simulink model "Proyecto_Final"  (R2017a)
settings: Solver=ode45  StartTime=0.0  StopTime=inf  FixedStep=0.002  RelTol=1e-4
values from neighbouring files (symbols this model uses):
  b_h = b_eq_h * r_h ^ 2 / R_d ^ 2    (= 28800)    [automatas_matlab.m]
  b_t = b_eq_t * r_t ^ 2 / R_w_t ^ 2    (= 27000)    [automatas_matlab.m]
  b_w_h = 30000    [automatas_matlab.m]
  ba_h = M_h * n_h * w_pos_h    (= 172800)    [automatas_matlab.m]
  ba_t = M_t * n_t * w_pos_t    (= 135000)    [automatas_matlab.m]
  bottom_limit_0 = -22    [automatas_matlab.m]
  bottom_limit_1 = -20    [automatas_matlab.m]
  container_vector = [2, 6, 4, 1, 5, 8, 1, 3, 7, 1, 5, 6]    [automatas_matlab.m]    (also in plot_crane.m = [8, 12, 12, 4, 5, 8, 1, 3]; test_traj.m = [8, 5, 9, 4, 5, 8, 4, 6]; test_trajectories.m = [8, 12, 12, 4, 5, 8, 1, 3, 7, 1, 5, 6])
  g = 9.80665    [automatas_matlab.m]
  h_contenedor = 2.79    [automatas_matlab.m]
  K_w_h = 1800000    [automatas_matlab.m]
  Ksa_h = M_h * n_h * w_pos_h^2    (= 207298.578199)    [automatas_matlab.m]
  Ksa_t = M_t * n_t * w_pos_t^2    (= 123542.570499)    [automatas_matlab.m]
  Ksia_h = M_h * w_pos_h ^ 3    (= 82894.8698367)    [automatas_matlab.m]
  Ksia_t = M_t * w_pos_t ^ 3    (= 45223.0125199)    [automatas_matlab.m]
  lambda = 0.91    [automatas_matlab.m]
  left_limit_0 = -32    [automatas_matlab.m]
  left_limit_1 = -30    [automatas_matlab.m]
  M_h = (J_d + J_m_h * r_h ^ 2)/ R_d ^ 2    (= 48014.2222222)    [automatas_matlab.m]
  m_l = 65000    [automatas_matlab.m]
  m_l_min = 15000    [automatas_matlab.m]
  M_t = m_c + (J_w_t + J_m_t * r_t ^ 2)/ R_w_t ^ 2    (= 59008)    [automatas_matlab.m]
  R_d = 0.75    [automatas_matlab.m]
  r_h = 30    [automatas_matlab.m]
  r_t = 15    [automatas_matlab.m]
  R_w_t = 0.5    [automatas_matlab.m]
  right_limit_0 = 52    [automatas_matlab.m]
  right_limit_1 = 50    [automatas_matlab.m]
  top_limit_0 = 42    [automatas_matlab.m]
  top_limit_1 = 40    [automatas_matlab.m]
  v_max_h_load = 1.5    [automatas_matlab.m]
  v_max_h_unload = 3    [automatas_matlab.m]
  v_max_t = 4    [automatas_matlab.m]
  x_t0 = 0    [automatas_matlab.m]
  y_t0 = 45    [automatas_matlab.m]    (also in crane.m; plot_crane.m; plot_crane_test.m)
  yl0 = h_contenedor + 5    (= 7.79)    [automatas_matlab.m]
undefined symbols (not defined in the file or in its folder): DiscIntNeverNeededParam
libraries: simulink x8, vrlib x1, sldrtlib x1
(part 2 of 2)

== stateflow chart Proyecto_Final/Level_1  ==
  settings: updateMethod=DISCRETE  sampleTime=0.01
  state Level1
    entry:
    go_to_ship = 1;
    to_manual = 0;
    ml = m_l;
    v_max_h = v_max_h_load;
    charged = 1;
    during:
    state Start [parallel]
      entry:
      traj_plt = plot(0, 0, 'r' );
      during:
      settings: executionOrder=4
      state Automatico
        entry:
        pos_ini_ = pos_ini;
        pos_fin_ = pos_fin;
        if go_to_ship == 0
        [pos_ini_, pos_fin_] = get_pos(pos_ini, pos_fin, container_vector);
        end
        [x_traj, y_traj] = get_trajectories(pos_ini_, pos_fin_, charged, container_vector);
        mode = 0;
        hold on
        during:
        %v_h_1 = 0.1;
        %v_t_1 = 0.1;
        state to_ship
          entry:
          to_ship_finished = 0;
          above_trajectory = 0;
          during:
          state Vertical
            entry:
            y_finish = get_y_finish();
            during:
            if y_finish > yl
            v_h_1 = - v_max_h * vertical_gain() ;
            else
            above_trajectory = 1;
            end
            v_t_1 = 0;
          state Diagonal_Up
            entry:
            [vh1_, vt1_] = get_v_up(1, 1);
            during:
            my_gain = get_gains();
            v_h_1 = vh1_ * my_gain;
            v_t_1 = vt1_ * my_gain;
          state Horizontal
            entry:
            during:
            my_gain = get_gains();
            v_h_1 = 0;
            v_t_1 = v_max_t * my_gain;
          state Diagonal_Down
            entry:
            [vh_1, vt_1] = get_v_down(1, 1);
            during:
            my_gain = get_gains();
            v_h_1 = vh_1 * my_gain;
            v_t_1 = vt_1 * my_gain;
          state Stop
            during:
            v_h_1 = 0;
            v_t_1 = 0;
            to_ship_finished = 1;
            go_to_ship = 0;
          (default) -> Level1.Start.Automatico.to_ship.Vertical
          Level1.Start.Automatico.to_ship.Vertical -> Level1.Start.Automatico.to_ship.Diagonal_Up [order 3] : [above_trajectory == 1]
          Level1.Start.Automatico.to_ship.Vertical -> Level1.Start.Automatico.to_ship.Diagonal_Down [order 2] : [xl > x_traj(3)]
          Level1.Start.Automatico.to_ship.Vertical -> Level1.Start.Automatico.to_ship.Diagonal_Up [order 1] : [(yl > (y_finish - 0.1)) && (yl < (y_finish + 0.1))]
          Level1.Start.Automatico.to_ship.Diagonal_Up -> Level1.Start.Automatico.to_ship.Horizontal : [yl >=  y_traj(2)]
          Level1.Start.Automatico.to_ship.Horizontal -> Level1.Start.Automatico.to_ship.Diagonal_Down : [xt > x_traj(3)]
          Level1.Start.Automatico.to_ship.Diagonal_Down -> Level1.Start.Automatico.to_ship.Stop : [xt > x_traj(4) && abs(yl - y_traj(4)) < 2]
        state from_ship
          entry:
          from_ship_finished = 0;
          above_trajectory = 0;
          during:
          state Vertical
            entry:
            y_finish = get_y_finish();
            during:
            if y_finish > yl
            v_h_1 = - v_max_h * vertical_gain();
            else
            above_trajectory = 1;
            end
            v_t_1 = 0;
          state Diagonal_Up
            entry:
            [vh1_, vt1_] = get_v_up_return(1, 1);
            during:
            my_gain = get_gains_return();
            v_h_1 = vh1_ * my_gain;
            v_t_1 = vt1_ * my_gain;
          state Horizontal
            entry:
            during:
            my_gain = get_gains_return();
            v_h_1 = 0;
            v_t_1 = -v_max_t * my_gain;
          state Diagonal_Down
            entry:
            [vh_1, vt_1] = get_v_down_return(1, 1);
            during:
            my_gain = get_gains_return();
            v_h_1 = vh_1 * my_gain;
            v_t_1 = vt_1 * my_gain;
          state Stop
            during:
            v_h_1 = 0;
            v_t_1 = 0;
            from_ship_finished = 1;
            go_to_ship = 1;
          (default) -> Level1.Start.Automatico.from_ship.Vertical
          Level1.Start.Automatico.from_ship.Vertical -> Level1.Start.Automatico.from_ship.Diagonal_Up [order 3] : [above_trajectory == 1]
          Level1.Start.Automatico.from_ship.Vertical -> Level1.Start.Automatico.from_ship.Diagonal_Down [order 2] : [xl < x_traj(2)]
          Level1.Start.Automatico.from_ship.Vertical -> Level1.Start.Automatico.from_ship.Diagonal_Up [order 1] : [(yl > (y_finish - 0.1)) && (yl < (y_finish + 0.1))]
          Level1.Start.Automatico.from_ship.Diagonal_Up -> Level1.Start.Automatico.from_ship.Horizontal : [yl >=  y_traj(3)]
          Level1.Start.Automatico.from_ship.Horizontal -> Level1.Start.Automatico.from_ship.Diagonal_Down : [xt < x_traj(2)]
          Level1.Start.Automatico.from_ship.Diagonal_Down -> Level1.Start.Automatico.from_ship.Stop : [xt < x_traj(1) && abs(yl - y_traj(1)) < 2]
        state Wait
          entry: from_ship_finished = 0;
          to_ship_finished = 0;
          entry:
          during:
          v_h_1 = 0;
          v_t_1 = 0;
        (default) -> Wait
        Wait -> from_ship [order 2] : [go_to_ship == 0 && automatic == 1]
        Wait -> to_ship [order 1] : [go_to_ship == 1 && automatic == 1]
        from_ship -> Wait : [from_ship_finished == 1 || go_to_ship == 1]
        to_ship -> Wait : [to_ship_finished == 1 || go_to_ship == 0]
      state Manual
        entry:
        %set(traj_plt, 'Visible', 'off')
        to_manual = 0;
        mode = 1;
        during:
        v_t_1 = calculate_vt1();
        v_h_1 = calculate_vh1();
      state Finales_carrera
        during:
        if bottom_limit == 1 || top_limit == 1
        v_t_1 = calculate_vt1();
        v_h_1 = 0;
        end
        if right_limit == 1 || left_limit == 1
        v_t_1 = 0;
        v_h_1 = calculate_vh1();
        end
      (default) -> Automatico
      Manual -> Automatico [order 1] : [automatic == 1 && after(1, sec) && yl > get_automatic_high()]
      Automatico -> Manual [order 2] : [abs(V_t_joystick) > 0.5  || abs(V_h_joystick > 0.5)]
      Automatico -> Manual [order 3] : [to_manual == 1]
      Finales_carrera -> Manual : [bottom_limit == 0 && top_limit == 0 && left_limit == 0 && right_limit == 0 ]
      Manual -> Finales_carrera [order 2] : [bottom_limit == 1 || top_limit == 1 || left_limit == 1 || right_limit == 1 ]
      Automatico -> Finales_carrera [order 1] : [bottom_limit == 1 || top_limit == 1 || left_limit == 1 || right_limit == 1 ]
    state Spreader [parallel]
      settings: executionOrder=1
      state Charged
        during:
        ml = m_l;
        v_max_h = v_max_h_load;
        charged = 1;
      state Unchaged
        during:
        ml = m_l_min;
        v_max_h = v_max_h_unload;
        charged = 0;
      (default) -> Charged
      Charged -> Unchaged : [twistlocks == 0]
      Unchaged -> Charged : [twistlocks == 1]
    state GUI [parallel]
      during:
      if submitGUI == 1
      to_manual = 1;
      go_to_ship = cons_to_ship;
      [x_traj, y_traj] = get_trajectories(pos_ini_, pos_fin_, charged, container_vector);
      else
      to_manual = 0;
      end
      settings: executionOrder=5
    state Balancing_Control [parallel]
      settings: executionOrder=2
      state Activated
        during:
        balancing = 1;
      state Disactivated
        during:
        balancing = 0;
      (default) -> Activated
      Activated -> Disactivated : [balancing_control == 1 && after(1, sec)]
      Disactivated -> Activated : [balancing_control == 1 && after(1, sec)]
    state Singal_ok [parallel]
      settings: executionOrder=3
      state On
        during:
        signal_ok = 1;
      state Off
        during:
        signal_ok = 0;
      (default) -> On
      On -> Off : after(1,sec)
      Off -> On : after(1,sec)
  (default) -> Level1
  data: vgain function_output; high function_output; vt1 function_output; vh1 function_output; ini function_input; fin function_input; x_points_trap function_output; y_points_trap function_output; charged_container function_input; containers function_input; vh1 function_output; vt1 function_output; gain_larger_x function_input; gain_larger_y function_input; yfinish function_output; vh1 function_output; vt1 function_output; gain_larger_x function_input; gain_larger_y function_input; vh1 function_output; vt1 function_output; gain_larger_x function_input; gain_larger_y function_input; vh1 function_output; vt1 function_output; gain_larger_x function_input; gain_larger_y function_input; gain function_output; gain function_output; ini function_input; fin function_input; my_ini function_output; my_fin function_output; containers function_input; xl input; yl input; xt input; V_t_joystick input; V_h_joystick input; automatic input; balancing_control input; twistlocks input; v_h_1 output; v_t_1 output; signal_ok output; balancing output; ml output; m_l input double; m_l_min input double; v_max_t input; v_max_h_unload input; v_max_h_load input; v_max_h local; charged output; mode output; bottom_limit input; top_limit input; left_limit input; right_limit input; pos_fin input; pos_ini input; traj_plt local; y_finish local; vh1_ local; vt1_ local; vh_1 local; vt_1 local; from_ship_finished local; to_ship_finished local; above_trajectory local; go_to_ship local; my_gain local; pos_fin_ local; pos_ini_ local; container_vector input; x_traj output; y_traj output; cons_to_ship input; submitGUI input; to_manual local
  function vgain = vertical_gain:
    | function vgain = vertical_gain
    |  v_gain = 1;
    | if abs(yl - y_finish) < 1
    |     vgain = 0.25;
    | else
    |     if abs(yl - y_finish) < 4
    |         vgain = 0.5;
    |     else
    |         vgain = 1;
    |     end
    | end
  function high = get_automatic_high:
    | function high = get_automatic_high
    |  
    | [x_traj, y_traj] = get_trajectories(pos_ini_, pos_fin_, charged, container_vector);
    | 
    | if (xl < 0)
    |     high = y_traj(1);
    | else
    |     high = y_traj(4);
    | end
  function vt1 = calculate_vt1:
    | function vt1 = calculate_vt1
    |  security_factor = 0.7;
    | if (abs(V_t_joystick) > 0.5)
    |     vt1 = v_max_t * security_factor * V_t_joystick;
    | else
    |     vt1 = 0;
    | end
    | end
  function vh1 = calculate_vh1:
    | function vh1 = calculate_vh1
    | security_factor = 0.7;
    | if (abs(V_h_joystick) > 0.5)
    |     vh1 = security_factor * v_max_h * V_h_joystick;
    | else
    |     vh1 = 0;
    | end
    | end
  function [x_points_trap, y_points_trap] = get_trajectories(ini, fin, charged_container, containers):
    | function [x_points_trap, y_points_trap] = get_trajectories(ini, fin, charged_container, containers)
    | 
    | to_ship = 1;
    | [x_points_trap, y_points_trap] = traj_trapezoid(ini, fin, charged_container, containers, to_ship);
    | 
    | end
  function [vh1, vt1] = get_v_down(gain_larger_x, gain_larger_y):
    | function [vh1, vt1] = get_v_down(gain_larger_x, gain_larger_y)
    |  
    | distance_x = abs(xl - x_traj(4));
    | distance_y = abs(yl - y_traj(4));
    | 
    | if distance_y > distance_x
    |     vh1 = gain_larger_y * v_max_h;
    |     vt1 = gain_larger_y * v_max_h * distance_x /distance_y;
    | else
    |     vt1 = v_max_t;
    |     vh1 = v_max_t * distance_y /distance_x;
    |     
    |     if vh1 > v_max_h
    |         r = vh1 / v_max_h;
    |         vt1 = vt1 / r;
    |         vh1 = vh1 / r;
    |     end
    |     vt1 = gain_larger_x * vt1;
    |     vh1 = gain_larger_y * vh1;
    | end
    | 
    | end
  function yfinish = get_y_finish:
    | function yfinish = get_y_finish()
    | 
    | yfinish = 45;
    | 
    | for i=1:length(x_traj)
    |     value = 1;
    |     if xl < x_traj(1)
    |         yfinish = y_traj(1);
    |         break;
    |     end
    |     if xl > x_traj(4)
    |         yfinish = y_traj(4);
    |     end
    |     if xl < x_traj(i)
    |         yfinish = (y_traj(i) - y_traj(i - 1)) / (x_traj(i) - x_traj(i - 1)) * (xl - x_traj(i - 1)) + y_traj(i - 1);
    |         break
    |     end
    | end
    |         
    | end
  function [vh1, vt1] = get_v_up(gain_larger_x, gain_larger_y):
    | function [vh1, vt1] = get_v_up(gain_larger_x, gain_larger_y)
    | 
    | distance_x = abs(xl - x_traj(2));
    | distance_y = abs(yl - y_traj(2));
    | 
    | if distance_y > distance_x
    |     vh1 = - gain_larger_y * v_max_h;
    |     vt1 = gain_larger_y * v_max_h * distance_x /distance_y;
    | else
    |     vt1 = v_max_t;
    |     vh1 = -v_max_t * distance_y /distance_x;
    |     
    |     if vh1 > v_max_h
    |         r = vh1 / v_max_h;
    |         vt1 = vt1 / r;
    |         vh1 = vh1 / r;
    |     end
    |     vt1 = gain_larger_x * vt1;
    |     vh1 = gain_larger_y * vh1;
    | end
    | 
    | end
  function [vh1, vt1] = get_v_down_return(gain_larger_x, gain_larger_y):
    | function [vh1, vt1] = get_v_down_return(gain_larger_x, gain_larger_y)
    |  
    | distance_x = abs(xl - x_traj(1));
    | distance_y = abs(yl - y_traj(1));
    | 
    | 
    | if distance_y > distance_x
    |     vh1 = gain_larger_y * v_max_h;
    |     vt1 = - gain_larger_y * v_max_h * distance_x /distance_y;
    | else
    |     vt1 = - v_max_t;
    |     vh1 = v_max_t * distance_y /distance_x;
    |     
    |     if vh1 > v_max_h
    |         r = vh1 / v_max_h;
    |         vt1 = vt1 / r;
    |         vh1 = vh1 / r;
    |     end
    |     vt1 = gain_larger_x * vt1;
    |     vh1 = gain_larger_y * vh1;
    | end
    | 
    | end
  function [vh1, vt1] = get_v_up_return(gain_larger_x, gain_larger_y):
    | function [vh1, vt1] = get_v_up_return(gain_larger_x, gain_larger_y)
    | 
    | distance_x = abs(xl - x_traj(3));
    | distance_y = abs(yl - y_traj(3));
    | 
    | if distance_y > distance_x
    |     vh1 = - gain_larger_y * v_max_h;
    |     vt1 = - gain_larger_y * v_max_h * distance_x /distance_y;
    | else
    |     vt1 = - v_max_t;
    |     vh1 = -v_max_t * distance_y /distance_x;
    |     
    |     if vh1 > v_max_h
    |         r = vh1 / v_max_h;
    |         vt1 = vt1 / r;
    |         vh1 = vh1 / r;
    |     end
    |     vt1 = gain_larger_x * vt1;
    |     vh1 = gain_larger_y * vh1;
    | end
    | 
    | end
  function gain = get_gains:
    | function gain = get_gains()
    | gain = 1;
    | if abs(xl - x_traj(4)) > 100
    |     gain = 1;
    | else
    |     gain = 0.12 + 0.88 * abs(xt - x_traj(4)) / 100.0;
    | %    gain = 1;
    | % elseif abs(xl - x_traj(4)) > 15
    | %     gain = 1/2;
    | % elseif abs(xl - x_traj(4)) > 10
    | %     gain = 1/4;
    | % elseif abs(xl - x_traj(4)) > 5
    | %     gain = 1/4;
    | % elseif abs(xl - x_traj(4)) > 3
    | %     gain = 1/4;
    | % else
    | %     gain = 1/4;
    | end
    | 
    | end
  function gain = get_gains_return:
    | function gain = get_gains_return
    | % gain = 1;
    | % if abs(xl - y_traj(1)) > 20
    | %    gain = 1;
    | % elseif abs(xl - x_traj(1)) > 15
    | %     gain = 1/2;
    | % elseif abs(xl - x_traj(1)) > 10
    | %     gain = 1/4;
    | % elseif abs(xl - x_traj(1)) > 5
    | %     gain = 1/4;
    | % elseif abs(xl - x_traj(1)) > 3
    | %     gain = 1/4;
    | % else
    | %     gain = 1/4;
    | % end
    | gain = 1;
    | if abs(xl - x_traj(1)) > 100
    |     gain = 1;
    | else
    |     gain = 0.12 + 0.88 * abs(xt - x_traj(1)) / 100.0;
    | %    gain = 1;
    | % elseif abs(xl - x_traj(4)) > 15
    | %     gain = 1/2;
    | % elseif abs(xl - x_traj(4)) > 10
    | %     gain = 1/4;
    | % elseif abs(xl - x_traj(4)) > 5
    | %     gain = 1/4;
    | % elseif abs(xl - x_traj(4)) > 3
    | %     gain = 1/4;
    | % else
    | %     gain = 1/4;
    | end
    | 
    | end
  function [my_ini, my_fin]  = get_pos(ini, fin, containers):
    | function [my_ini, my_fin]  = get_pos(ini, fin, containers)
    | x_edge = 2;
    | y_edge = 2;
    | container_size_x = 2.44;
    | container_size_y = 2.79;
    | y_ini = 4;
    | y_platform = 0;
    | y_ship_botton = -10;
    | 
    | y_safe = 2;
    | 
    | position_vector = zeros(length(containers));
    | for i = 1:length(containers)
    |     position_vector(i) = i;
    | end
    | 
    | x_ini = 0;
    | y_fin = 0;
    | x_positions = position_vector * container_size_x - container_size_x / 2 + x_edge;
    | 
    | my_ini = ini;
    | my_fin = fin;
    | if xl > 0
    |     if xl > x_positions(length(x_positions))
    |         my_fin = length(x_positions);
    |     else
    |         for i = 1:length(x_positions)
    |             if xl < x_positions(i)
    |                 my_fin = i;
    |                 break;
    |             end
    |         end
    |     end
    | end
    |         
    |         
    |     
    |     
    |     
    | end

== stateflow chart Proyecto_Final/Chart ==
  settings: updateMethod=DISCRETE  sampleTime=0.3
  state Plotting
    state plot_structure
      entry:
      plot_crane(container_vector);
      tr_plt = rectangle('Position', [0,0,0,0], 'FaceColor',[1 1 1], 'EdgeColor','r','LineWidth',0.3);
      spr_plt = rectangle('Position', [0,0,0,0], 'FaceColor',[1 1 1], 'EdgeColor','r','LineWidth',0.3);
      wire_plt = plot([0,0],[0,0], 'r','linewidth', 3);
      ch_plt =  rectangle('Position', [0,0,0,0], 'FaceColor',[1 1 1], 'EdgeColor','r','LineWidth',0.3);
      tra_plt = plot([0,0,0,0],[0,0,0,0]);
      during:
      plot_trolley(xt);
      plot_spreader(xl, yl);
      plot_wire(xl, yl, xt);
      plot_indicators();
      plot_charged(xl, yl, charged);
      update_crane()
      set(tra_plt,'Visible','off')
      tra_plt = plot(x_traj, y_traj, 'r')
    state update_plt
      entry:
      update_crane()
    (default) -> plot_structure
    plot_structure -> update_plt : [update == 1]
    update_plt -> plot_structure : [update == 0]
  (default) -> Plotting
  data: containers function_input; xt_ function_input; xl_ function_input; yl_ function_input; xl_ function_input; yl_ function_input; xt_ function_input; xl_ function_input; yl_ function_input; charged_container function_input; xl input; yl input; xt input; balancing input; mode input; tr_plt local; spr_plt local; wire_plt local; charged input; emergency input; ch_plt local; update input; container_vector input; x_traj input; y_traj input; tra_plt local
  function plot_crane(containers):
    | function plot_crane(containers)
    | x_edge = 2;
    | y_edge = 2;
    | container_size_x = 2.44;
    | container_size_y = 2.79;
    | y_ini = 4;
    | y_platform = 0;
    | y_ship_bottom = -10;
    | y_safe = 2;
    | y_t0 = 45;
    | distancia_carriles = 1;
    | 
    | x_ini = 0;
    | y_fin = 0;
    | 
    | barco_extremo_der = length(containers) * container_size_x + x_edge + 0.5;
    | 
    | x_min = -36;
    | x_max = 56;
    | y_min = -25;
    | y_max = 50;
    | 
    | %Viga horizontal
    | Yvigah = [y_t0, y_t0];
    | Xvigah = [x_min x_max];
    | 
    | figure(1)
    | plot(Xvigah, Yvigah,'r','linewidth', 2)
    | 
    | 
    | 
    | xlim([x_min x_max])
    | ylim([y_min y_max])
    | hold on
    | % Muelle
    | 
    | Xmuelleh = [x_min, 0];
    | Ymuelleh = [0, 0];
    | Xmuellev = [0, 0];
    | Ymuellev = [0, y_ship_bottom];
    | 
    | plot(Xmuelleh, Ymuelleh, 'k','linewidth', 3)
    | plot(Xmuellev, Ymuellev, 'k','linewidth', 3)
    | 
    | %Barco
    | 
    | Ybarco_izq = [y_edge, y_ship_bottom];
    | Xbarco_izq = [x_edge - 0.5 , x_edge - 0.5];
    | 
    | Ybarco_abajo = [y_ship_bottom - 0.2, y_ship_bottom - 0.3];
    | Xbarco_abajo = [x_edge - 0.8, barco_extremo_der + 0.3];
    | 
    | 
    | 
    | Ybarco_der = [y_edge, y_ship_bottom];
    | Xbarco_der = [barco_extremo_der, barco_extremo_der ];
    | 
    | plot(Xbarco_izq, Ybarco_izq, 'r','linewidth', 3)
    | plot(Xbarco_abajo, Ybarco_abajo, 'r','linewidth', 3)
    | plot(Xbarco_der, Ybarco_der, 'r','linewidth', 3)
    | 
    | 
    | position_vector = zeros(length(containers));
    | for i = 1:length(containers)
    |     position_vector(i) = i;
    | end
    | 
    | x_positions = position_vector * container_size_x - container_size_x + x_edge ;
    | 
    | for i = 1:length(containers)
    |     center_container_y = 0 + y_ship_bottom;
    |     for j = 1:containers(i)
    |         
    |         rectangle('Position', [x_positions(i),center_container_y, container_size_x, container_size_y], 'FaceColor',[0.5 0.5 0.5], 'EdgeColor','k','LineWidth',0.3)
    |         center_container_y = center_container_y + container_size_y;
    |     end
    | end
    | 
    | distancia_carriles = 4;
    | containers2 = [1, 1, 1];
    | x_positions2 = [0 0 0];
    | x_positions2(1) = -3 * distancia_carriles - container_size_x/2;
    | x_positions2(2) = -2 * distancia_carriles - container_size_x/2;
    | x_positions2(3) = -1 * distancia_carriles - container_size_x/2;
    | 
    | 
    | 
    | for i = 1:length(containers2 )
    |     center_container_y = 0;
    |     for j = 1:containers2(i)
    |         
    |         rectangle('Position', [x_positions2(i),center_container_y, container_size_x, container_size_y], 'FaceColor',[0.5 0.5 0.5], 'EdgeColor','k','LineWidth',0.3)
    |         center_container_y = center_container_y + container_size_y;
    |     end
    | end
    | 
    | % Marcadores de formas de funcionamiento
    | x_text = -30;
    | y_text = -10;
    | txt = 'Level 0';
    | text(x_text, y_text + 3, txt);
    | txt = 'Manual';
    | text(x_text, y_text, txt);
    | txt = 'Charged';
    | text(x_text, y_text - 3, txt);
    | txt = 'Balancing Control';
    | text(x_text, y_text - 6, txt);
    | 
    | 
    | 
    | 
    | end
  function plot_trolley(xt_):
    | function plot_trolley(xt_)
    | %delete(tr_plt);
    | set(tr_plt,'Visible','off')
    | trolley_size_x = 4;
    | trolley_size_y = 2.5;
    | trolley_y = 45;
    | trolley_x = xt_ - trolley_size_x / 2;
    | tr_plt = rectangle('Position', [trolley_x, trolley_y, trolley_size_x, trolley_size_y], 'FaceColor',[1 1 1], 'EdgeColor','r','LineWidth',0.3);
    | end
  function plot_spreader(xl_, yl_):
    | function plot_spreader(xl_, yl_)
    | 
    | set(spr_plt,'Visible','off')
    | 
    | spreader_size_x = 0.4;
    | spreader_size_y = 0.4;
    | 
    | 
    | spr_plt = rectangle('Position', [xl_ - spreader_size_x/2, yl_ - spreader_size_y/2, spreader_size_x, spreader_size_y], 'FaceColor',[0 0 0], 'EdgeColor','k','LineWidth',0.3);
    | 
    | end
  function plot_wire(xl_, yl_, xt_):
    | function plot_wire(xl_, yl_, xt_)
    | 
    | set(wire_plt,'Visible','off')
    | x_trolley = xt_; 
    | y_trolley = 45;
    | x_spreader = xl_;
    | y_spreader = yl_;
    | 
    | point_trolley = [x_trolley, x_spreader];
    | point_spreader = [y_trolley, y_spreader];
    | 
    | wire_plt = plot(point_trolley,point_spreader, 'k','linewidth', 1.5);
    | end
  function plot_indicators:
    | function plot_indicators()
    | x_circle = -5;
    | y_circles = -10 - 1;
    | if emergency == 0
    |     rectangle('Position', [x_circle, y_circles + 3, 2, 2], 'FaceColor',[1 0 0], 'EdgeColor','r','LineWidth',0.3);
    | else
    |     rectangle('Position', [x_circle, y_circles + 3, 2, 2], 'FaceColor',[0 1 0], 'EdgeColor','g','LineWidth',0.3);
    | end
    | 
    | if mode == 0
    |      rectangle('Position', [x_circle, y_circles, 2, 2], 'FaceColor',[1 0 0], 'EdgeColor','r','LineWidth',0.3);
    | else
    |     rectangle('Position', [x_circle, y_circles, 2, 2], 'FaceColor',[0 1 0], 'EdgeColor','g','LineWidth',0.3);
    | end
    | 
    | if charged == 0
    |     rectangle('Position', [x_circle, y_circles - 3, 2, 2], 'FaceColor',[1 0 0], 'EdgeColor','r','LineWidth',0.3);
    | else
    |     rectangle('Position', [x_circle, y_circles - 3, 2, 2], 'FaceColor',[0 1 0], 'EdgeColor','g','LineWidth',0.3);
    | end
    | 
    | if balancing == 0
    |     rectangle('Position', [x_circle, y_circles - 6, 2, 2], 'FaceColor',[1 0 0], 'EdgeColor','r','LineWidth',0.3);
    | else
    |     rectangle('Position', [x_circle, y_circles - 6, 2, 2], 'FaceColor',[0 1 0], 'EdgeColor','g','LineWidth',0.3);
    | end
    | 
    | end
  function plot_charged(xl_, yl_, charged_container):
    | function plot_charged(xl_, yl_, charged_container)
    | container_size_x = 2.44;
    | container_size_y = 2.79;
    | if charged_container == 0
    |     set(ch_plt,'Visible','off');
    | end
    | if charged_container == 1
    |     set(ch_plt,'Visible','off');
    |     center_container_x = xl_ - container_size_x / 2;
    |     center_container_y = yl_ - container_size_y;
    |     ch_plt = rectangle('Position', [center_container_x, center_container_y, container_size_x, container_size_y], 'FaceColor',[0.5 0.5 0.5], 'EdgeColor','k','LineWidth',0.3);
    | end
    | end
  function update_crane:
    | function update_crane
    | if update == 1 
    |     clf(1, 'reset')
    | end
    | end

== stateflow chart Proyecto_Final/Controller/Chart ==
  state Up
    during:
    output = 1;
  state Down
    during:
    output = 0;
  (default) -> Up
  Up -> Down : [input == 1 && after(1, sec)]
  Down -> Up : [input == 1 && after(1, sec)]
  data: output output; input input

== matlab function Proyecto_Final/controller-plant1/Controlador/Subsystem1/Control de angulo 1/MATLAB Function ==
  data: lh input; kp output; m input; p input; Mt input; bt input; kd output
function [kp,kd] = fn(lh,m,p,Mt,bt)

kd =  lh - Mt * 9.81 / ((Mt + m) * (p^2));
kp = 2 * p * (lh - kd);

== matlab function Proyecto_Final/controller-plant1/Planta/Balanceo ==
  data: xl input; l output; yl input; xt0 input; yt0 input; tita output
function [l,tita] = fcn(xl,yl,xt0,yt0)

deltax = (xl - xt0);
deltay = -(yl - yt0);


l = sqrt((deltax ^ 2) + (deltay ^ 2));

tita = atan2(deltax, deltay);

end
